simulink model "power_battery_nimh_model_noncode"  (R2017a)
settings: Solver=ode23tb  StartTime=0.0  StopTime=7200  MaxStep=0.1  RelTol=1e-4  EnableMultiTasking=on
undefined symbols (not defined in the file): Hydride, Metal, Nickel
libraries: powerlib x7, electricdrivelib x1
Description:
  | Copyright 2008-2017 The MathWorks, Inc.
settings Model: Creator=MathWorks  LastModifiedBy=hlope
settings DataIOCC: LimitDataPoints=on  SaveFormat=Array
settings OptimizationCC: ExpressionDepthLimit=2147483647  InitFltsAndDblsToZero=on  LifeSpan=inf
settings DebuggingCC: UnderspecifiedInitializationDetection=Classic  MergeDetectMultiDrivingBlocksExec=none  SignalResolutionControl=TryResolveAllWithWarning  SolverPrmCheckMsg=warning  FcnCallInpInsideContextMsg=warning  AllowSymbolicDim=off  StateNameClashWarn=warning  SFUnexpectedBacktrackingDiag=warning  SFNoUnconditionalDefaultTransitionDiag=warning  SFExecutionAtInitializationDiag=none
settings HardwareCC: ProdBitPerPointer=32  ProdBitPerSizeT=32  ProdBitPerPtrDiffT=32  ProdLargestAtomicFloat=None  ProdIntDivRoundTo=Undefined  ProdEndianess=Unspecified  ProdWordSize=32  ProdHWDeviceType=32-bit Generic
settings ModelReferenceCC: PropagateSignalLabelsOutOfModel=off
settings GRTTargetCC: TargetLangStandard=C89/C90 (ANSI)  GeneratePreprocessorConditionals=Disable all  CombineOutputUpdateFcns=off  GRTInterface=on
settings ConfigComp: CovMetricSettings=dw  CovHtmlReporting=on  CovSaveCumulativeToWorkspaceVar=on  CovSaveSingleToWorkspaceVar=on  CovExternalEMLEnable=off

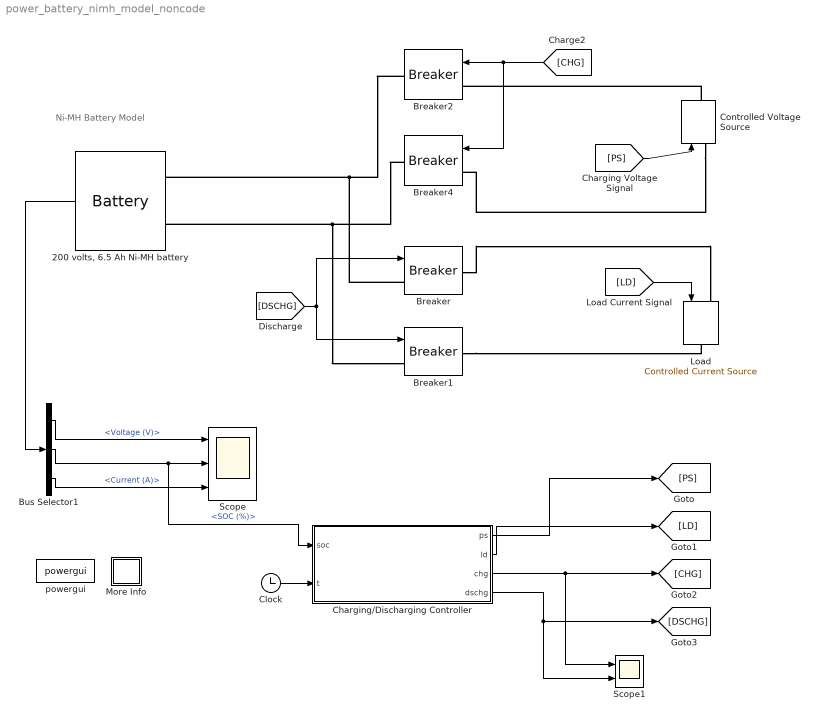
== system power_battery_nimh_model_noncode ==
  note: Ni-MH Battery Model
  "200 volts, 6.5 Ah Ni-MH battery " : electricdrivelib/Extra Sources/Battery  BatType=Nickel-Metal-Hydride  ShowTempParam=on  ThermalPreset=no  ShowAgeParam=off  NomV=200  NomQ=6.5  SOC=100  Batt_Tr=30  PresetModel=on  MaxQ=7  MinV=150  FullV=235.5932  Dis_rate=1.3  R=0.30769  Normal_OP=6.25  expZone="[216.9492           1.3]"  current=50  Units=Ampere-hour  Tci=20  NomT=25  T2=0  MaxQ2=2.208  FullV2=3.45  Normal_OP2=2.8  expZone2="[3.22        0.23]"  Rca=0.6  ti=1000  Dp=0  Neq0=0  Tsim=1e6  Ta1=25  Qeol=5.4*0.9  Reol=0.013333*1.2  Char_age=[2.3478, 3]  Dis_age=[2.3478, 10]  N1=1500  N2=10500  N3=1000  N4=1400  Ta2=45  N5=950
  Breaker{,1..2,4} (4 alike) : powerlib/Elements/Breaker  InitialState=0  SwitchingTimes="[1/60  5/60]"  External=on  BreakerResistance=0.01  SnubberResistance=1e6  SnubberCapacitance=inf  Measurements=None  MoreParameters=on  NoBreakLoop=off
      settings: SourceProductName=Simscape Power Systems
  Bus Selector1 : BusSelector  OutputSignals=Voltage (V),SOC (%),Current (A)
  Charging/Discharging Controller : MATLAB Function  TreatAsAtomicUnit=on
  Clock : Clock
  Controlled Voltage Source : powerlib/Electrical Sources/Controlled Voltage Source  Initialize=on  Source_Type=AC  Amplitude=0  Phase=0  Frequency=0  Measurements=None
  "Load " : powerlib/Electrical Sources/Controlled Current Source  Initialize=on  Source_Type=AC  Amplitude=0  Phase=0  Frequency=0  Measurements=None
  More Info : Subsystem
      settings: OpenFcn=showdemo(bdroot(gcb))
      mask Display: disp('?')
  Scope : Scope  NumInputPorts=3
  Scope1 : Scope  NumInputPorts=2
  powergui : powerlib/powergui  SimulationMode=Continuous  SampleTime=0.001  frequency=60  Iterations=50  frequencyindice=0  Pbase=100e6  ErrMax=1e-4  UnitsV=kV  UnitsW=MW  buscounter=0  FunctionMessages=off  echomessages=off  EnableUseOfTLC=off  CurrentSourceSwitches=off  DisableSnubberDevices=off  DisableRonSwitches=off  DisableVfSwitches=off  DisplayEquations=off  SolverType=Tustin  Interpol=off  ExternalGateDelay=off  methode=off  Ts=0  x0status=blocks  SPID=off  SwTol=0  HookPort=off  RestoreLinks=warning  ResistiveCurrentMeasurement=off  Frange=[0:2:500]  Ylog=off  Xlog=on  ShowGrid=off  save=off  variable=ZData  structure=0  ZoomFFT=on  StartTime=0.0  cycles=1  DisplayStyle=1  fundamental=60  FreqAxis=off  MaxFrequency=1000  frequencyindicesteady=1  RmsSteady=1  display=off
  wires:
  "200 volts, 6.5 Ah Ni-MH battery "/1 -> Bus Selector1/1
  Bus Selector1/2 -> Scope/2, Charging/Discharging Controller/1(soc)  "<SOC (%)>"
  Bus Selector1/1 -> Scope/1  "<Voltage (V)>"
  Bus Selector1/3 -> Scope/3  "<Current (A)>"
  Charging/Discharging Controller/1(ps) -> [PS]
  Charging/Discharging Controller/2(ld) -> [LD]
  Charging/Discharging Controller/3(chg) -> Scope1/1, [CHG]
  Charging/Discharging Controller/4(dschg) -> Scope1/2, [DSCHG]
  Clock/1 -> Charging/Discharging Controller/2(t)
  [PS] -> Controlled Voltage Source/1
  [CHG] -> Breaker4/1, Breaker2/1
  [DSCHG] -> Breaker1/1, Breaker/1
  [LD] -> "Load "/1
  connections:
  Breaker2/RConn1 -- Breaker/LConn1 -- "200 volts, 6.5 Ah Ni-MH battery "/LConn1
  Controlled Voltage Source/RConn1 -- Breaker2/LConn1
  Breaker4/RConn1 -- Breaker1/LConn1 -- "200 volts, 6.5 Ah Ni-MH battery "/LConn2
  Controlled Voltage Source/LConn1 -- Breaker4/LConn1
  Breaker1/RConn1 -- "Load "/RConn1
  Breaker/RConn1 -- "Load "/LConn1

== system power_battery_nimh_model_noncode/More Info ==

== matlab function power_battery_nimh_model_noncode/Charging//Discharging Controller ==
  data: ps output; ld output; soc input; chg output; dschg output; t input
function [ps, ld,chg, dschg] = fcn(soc,t)
% Create a charge/discharge condition
ps = 250;
ld = 6.5;
chg=0;dschg=0;

if( soc <= 40)
chg=1;
dschg=0;
else
    chg=0;
    dschg=1;
end

if( soc > 50)
  chg=0;
  dschg=0;
end


end
